simulink model "Vaja7b"  (R2013a)
settings: Solver=ode45  StartTime=0.0  StopTime=1  MaxStep=1e-4
undefined symbols (not defined in the file or in its folder): DiscIntNeverNeededParam
libraries: simulink x3
settings Model: Creator=Studenti  LastModifiedBy=Studenti
settings DataIOCC: SignalLoggingSaveFormat=ModelDataLogs
settings DebuggingCC: MaxConsecutiveZCsMsg=none  MultiTaskDSMMsg=warning  MultiTaskCondExecSysMsg=none  StrictBusMsg=None
settings RTWCC: IncludeERTFirstTime=on
settings GRTTargetCC: CodeReplacementLibrary=None  CPPClassGenCompliant=on

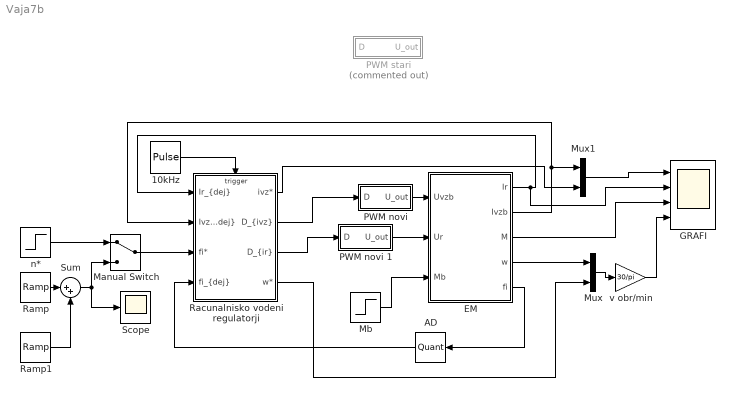
== system Vaja7b ==
  10kHz : DiscretePulseGenerator  PulseType=Time based  Period=1/10000  PulseWidth=5
  AD : Quantizer  QuantizationInterval=2*pi*2^-10
  EM : Subsystem  RequirementInfo="{}  %GIDa_e134c5b2_b96c_49ed_8b06_b6a8320c10d0"
  GRAFI : Scope  NumInputPorts=4
      settings: TimeRange=1  YMin=-4~0~-1~-100  YMax=4~0.5~1~300
  Manual Switch : ManualSwitch
  Mb : Step  Time=0.1  After=0.3  SampleTime=0
  Mux : Mux  Inputs=2
  Mux1 : Mux  Inputs=2
  "PWM novi " : Subsystem
  PWM novi 1 : Subsystem
  PWM stari : Subsystem  Commented=on
  Racunalnisko vodeni regulatorji : Subsystem
  Ramp : simulink/Sources/Ramp  slope=90*2*pi/60  start=0.1  X0=0
  Ramp1 : simulink/Sources/Ramp  slope=-90*2*pi/60  start=0.8  X0=0
  Scope : Scope
      settings: SaveName=ScopeData2
  Sum : Sum  Inputs=|++
  n* : Step  Time=0.2  After=pi*2  SampleTime=0
  v obr/min : Gain  Gain=30/pi
  wires:
  EM/3(M) -> GRAFI/3
  "PWM novi "/1(U_out) -> EM/1(Uvzb)
  PWM novi 1/1(U_out) -> EM/2(Ur)
  Mux/1 -> v obr/min/1
  Mb/1 -> EM/3(Mb)
  10kHz/1 -> Racunalnisko vodeni regulatorji/Trigger
  EM/2(Ivzb) -> Mux1/1, Racunalnisko vodeni regulatorji/2("Ivz_{dej}")
  Racunalnisko vodeni regulatorji/2("D_{ivz}") -> "PWM novi "/1(D)
  Racunalnisko vodeni regulatorji/1(ivz*) -> Mux1/2
  Racunalnisko vodeni regulatorji/3("D_{ir}") -> PWM novi 1/1(D)
  Racunalnisko vodeni regulatorji/4(w*) -> Mux/2
  EM/1(Ir) -> GRAFI/2, Racunalnisko vodeni regulatorji/1("Ir_{dej}")
  v obr/min/1 -> GRAFI/4
  EM/5(fi) -> AD/1
  AD/1 -> Racunalnisko vodeni regulatorji/4("fi_{dej}")
  EM/4(w) -> Mux/1
  Manual Switch/1 -> Racunalnisko vodeni regulatorji/3(fi*)
  n*/1 -> Manual Switch/1
  Ramp1/1 -> Sum/2
  Ramp/1 -> Sum/1
  Sum/1 -> Scope/1, Manual Switch/2
  Mux1/1 -> GRAFI/1

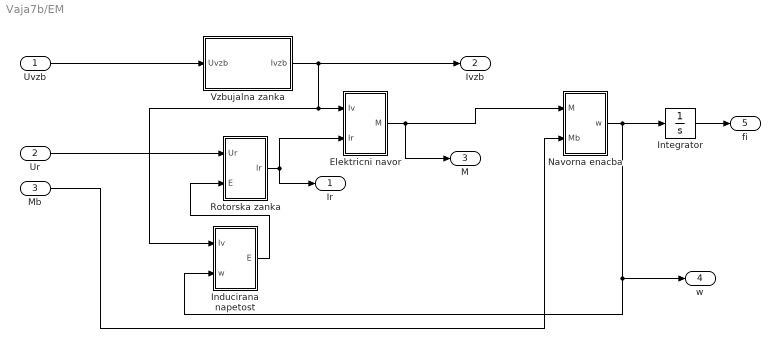
== system Vaja7b/EM ==
  Uvzb : Inport
  Ur : Inport  Port=2
  Mb : Inport  Port=3
  Elektricni navor : Subsystem
  Inducirana napetost : Subsystem
  Integrator : Integrator
  Navorna enacba : Subsystem
  Rotorska zanka : Subsystem
  Vzbujalna zanka : Subsystem
  Ir : Outport
  Ivzb : Outport  Port=2
  M : Outport  Port=3
  w : Outport  Port=4
  fi : Outport  Port=5
  wires:
  Uvzb/1 -> Vzbujalna zanka/1(Uvzb)
  Vzbujalna zanka/1(Ivzb) -> Ivzb/1, Inducirana napetost/1(Iv), Elektricni navor/1(Iv)
  Rotorska zanka/1(Ir) -> Elektricni navor/2(Ir), Ir/1
  Navorna enacba/1(w) -> w/1, Inducirana napetost/2(w), Integrator/1
  Elektricni navor/1(M) -> M/1, Navorna enacba/1(M)
  Inducirana napetost/1(E) -> Rotorska zanka/2(E)
  Ur/1 -> Rotorska zanka/1(Ur)
  Mb/1 -> Navorna enacba/2(Mb)
  Integrator/1 -> fi/1

== system Vaja7b/PWM novi  ==
  D : Inport
  Saturation : Saturate  UpperLimit=24  LowerLimit=-24
  Transfer Fcn : TransferFcn  Numerator=[24]  Denominator=[1/10000 1]
  U_out : Outport
  wires:
  Saturation/1 -> U_out/1
  Transfer Fcn/1 -> Saturation/1
  D/1 -> Transfer Fcn/1

== system Vaja7b/PWM novi 1 ==
  D : Inport
  Saturation : Saturate  UpperLimit=24  LowerLimit=-24
  Transfer Fcn : TransferFcn  Numerator=[24]  Denominator=[1/10000 1]
  U_out : Outport
  wires:
  Saturation/1 -> U_out/1
  Transfer Fcn/1 -> Saturation/1
  D/1 -> Transfer Fcn/1

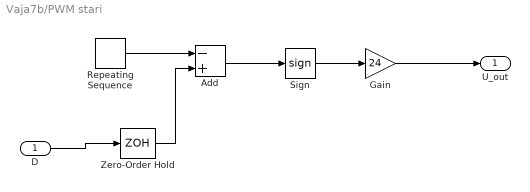
== system Vaja7b/PWM stari ==
  D : Inport
  Add : Sum  Inputs=-+
  Gain : Gain  Gain=24
  Repeating Sequence : simulink/Sources/Repeating Sequence  rep_seq_t=[0 0.0001]  rep_seq_y=[-1 1]
  Sign : Signum
  Zero-Order Hold : ZeroOrderHold  SampleTime=1/10000
  U_out : Outport
  wires:
  Gain/1 -> U_out/1
  Sign/1 -> Gain/1
  Repeating Sequence/1 -> Add/1
  Add/1 -> Sign/1
  Zero-Order Hold/1 -> Add/2
  D/1 -> Zero-Order Hold/1

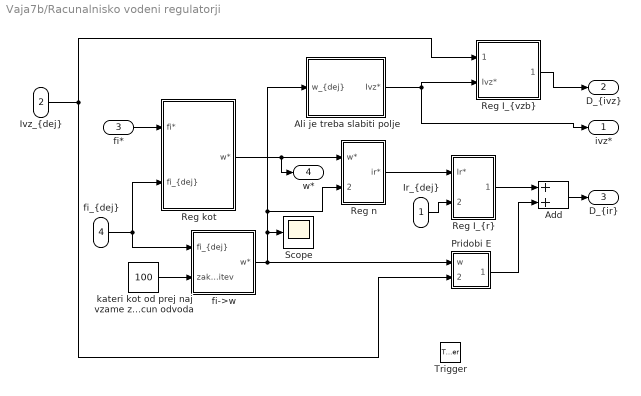
== system Vaja7b/Racunalnisko vodeni regulatorji ==
  "Ir_{dej}" : Inport
  "Ivz_{dej}" : Inport  Port=2
  fi* : Inport  Port=3
  "fi_{dej}" : Inport  Port=4
  Trigger : TriggerPort  PortDimensions=1
  Add : Sum
  Ali je treba slabiti polje : Subsystem
  Pridobi E : Subsystem
  "Reg I_{r}" : Subsystem
  "Reg I_{vzb}" : Subsystem
  Reg kot : Subsystem
  Reg n : Subsystem
  Scope : Scope
  fi->w : Subsystem
  kateri kot od prej naj vzame za izracun odvoda : Constant  Value=100
  ivz* : Outport
  "D_{ivz}" : Outport  Port=2
  "D_{ir}" : Outport  Port=3
  w* : Outport  Port=4
  wires:
  "Reg I_{r}"/1("D_{ir}") -> Add/1
  Reg n/1(ir*) -> "Reg I_{r}"/1(Ir*)
  "Reg I_{vzb}"/1("D_{ivz}") -> "D_{ivz}"/1
  Add/1 -> "D_{ir}"/1
  Ali je treba slabiti polje/1("Ivz* ") -> "Reg I_{vzb}"/2(Ivz*), ivz*/1
  Pridobi E/1(~E/24) -> Add/2
  Reg kot/1(w*) -> w*/1, Reg n/1(w*)
  "Ir_{dej}"/1 -> "Reg I_{r}"/2("Ir_{dej}")
  "Ivz_{dej}"/1 -> "Reg I_{vzb}"/1("Ivz_{dej}"), Pridobi E/2(Ivz)
  fi->w/1(w*) -> Scope/1, Ali je treba slabiti polje/1("w_{dej} "), Reg n/2("w_{dej}"), Pridobi E/1(w)
  "fi_{dej}"/1 -> fi->w/1("fi_{dej}"), Reg kot/2("fi_{dej}")
  kateri kot od prej naj vzame za izracun odvoda/1 -> fi->w/2(zakasnitev)
  fi*/1 -> Reg kot/1(fi*)

== system Vaja7b/EM/Elektricni navor ==
  Iv : Inport
  Ir : Inport  Port=2
  GQD : Gain  Gain=0.63
  Product : Product
  M : Outport
  wires:
  Ir/1 -> Product/2
  GQD/1 -> M/1
  Iv/1 -> Product/1
  Product/1 -> GQD/1

== system Vaja7b/EM/Inducirana napetost ==
  Iv : Inport
  w : Inport  Port=2
  GQD : Gain  Gain=0.63
  Product : Product
  E : Outport
  wires:
  Product/1 -> GQD/1
  Iv/1 -> Product/1
  w/1 -> Product/2
  GQD/1 -> E/1

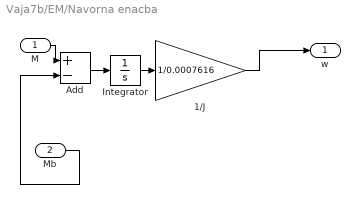
== system Vaja7b/EM/Navorna enacba ==
  M : Inport
  Mb : Inport  Port=2
  1/J : Gain  Gain=1/0.0007616
  Add : Sum  Inputs=+-
  Integrator : Integrator
  w : Outport
  wires:
  Integrator/1 -> 1/J/1
  1/J/1 -> w/1
  Add/1 -> Integrator/1
  M/1 -> Add/1
  Mb/1 -> Add/2

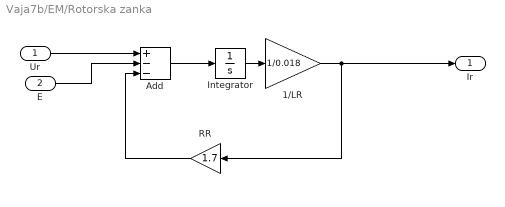
== system Vaja7b/EM/Rotorska zanka ==
  Ur : Inport
  E : Inport  Port=2
  1/LR : Gain  Gain=1/0.018
  Add : Sum  Inputs=+--
  Integrator : Integrator
  RR : Gain  Gain=1.7
  Ir : Outport
  wires:
  Add/1 -> Integrator/1
  Ur/1 -> Add/1
  RR/1 -> Add/3
  1/LR/1 -> RR/1, Ir/1
  Integrator/1 -> 1/LR/1
  E/1 -> Add/2

== system Vaja7b/EM/Vzbujalna zanka ==
  Uvzb : Inport
  1/Lv : Gain  Gain=1/4.01
  Integrator : Integrator
  Rv : Gain  Gain=25.8
  Sum : Sum  Inputs=|+-
  Ivzb : Outport
  wires:
  Rv/1 -> Sum/2
  Sum/1 -> Integrator/1
  Integrator/1 -> 1/Lv/1
  Uvzb/1 -> Sum/1
  1/Lv/1 -> Rv/1, Ivzb/1

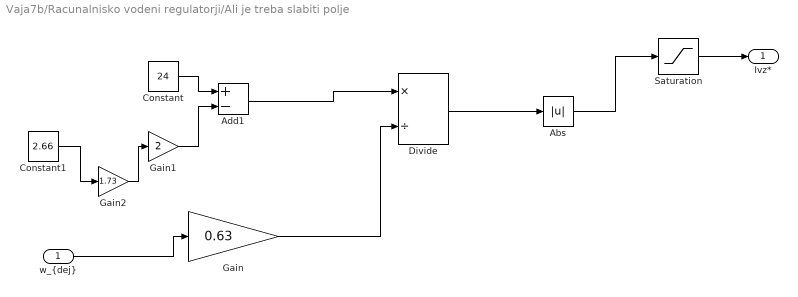
== system Vaja7b/Racunalnisko vodeni regulatorji/Ali je treba slabiti polje ==
  "w_{dej} " : Inport
  Abs : Abs
  Add1 : Sum  Inputs=+-
  Constant : Constant  Value=24
  Constant1 : Constant  Value=2.66
  Divide : Product  Inputs=*/
  Gain : Gain  Gain=0.63
  Gain1 : Gain  Gain=2
  Gain2 : Gain  Gain=1.73
  Saturation : Saturate  UpperLimit=0.48  LowerLimit=0
  "Ivz* " : Outport
  wires:
  Divide/1 -> Abs/1
  Saturation/1 -> "Ivz* "/1
  Gain1/1 -> Add1/2
  Abs/1 -> Saturation/1
  "w_{dej} "/1 -> Gain/1
  Gain/1 -> Divide/2
  Add1/1 -> Divide/1
  Constant/1 -> Add1/1
  Gain2/1 -> Gain1/1
  Constant1/1 -> Gain2/1

== system Vaja7b/Racunalnisko vodeni regulatorji/Pridobi E ==
  w : Inport
  Ivz : Inport  Port=2
  Divide : Product  Inputs=**
  Gain : Gain  Gain=0.63/24
  ~E/24 : Outport
  wires:
  Gain/1 -> ~E/24/1
  w/1 -> Divide/2
  Ivz/1 -> Divide/1
  Divide/1 -> Gain/1

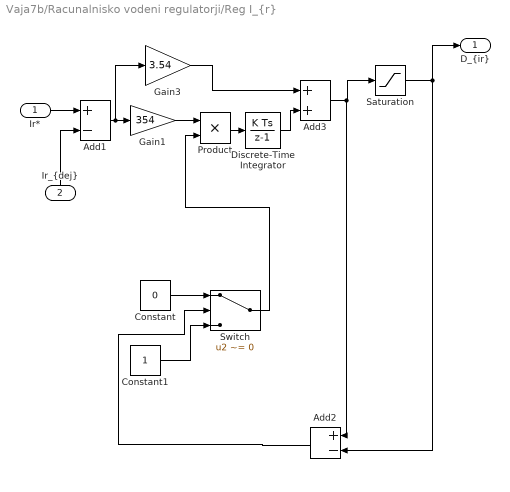
== system Vaja7b/Racunalnisko vodeni regulatorji/Reg I_{r} ==
  Ir* : Inport
  "Ir_{dej}" : Inport  Port=2
  Add1 : Sum  Inputs=+-
  Add2 : Sum  Inputs=+-
  Add3 : Sum
  Constant : Constant  Value=0
  Constant1 : Constant
  Discrete-Time Integrator : DiscreteIntegrator  SampleTime=-1  ICPrevOutput=DiscIntNeverNeededParam  ICPrevScaledInput=DiscIntNeverNeededParam
  Gain1 : Gain  Gain=354
  Gain3 : Gain  Gain=3.54
  Product : Product
  Saturation : Saturate  UpperLimit=1  LowerLimit=-1
  Switch : Switch  Criteria=u2 ~= 0  ZeroCross=off
  "D_{ir}" : Outport
  wires:
  Discrete-Time Integrator/1 -> Add3/2
  Gain3/1 -> Add3/1
  Add1/1 -> Gain1/1, Gain3/1
  "Ir_{dej}"/1 -> Add1/2
  Ir*/1 -> Add1/1
  Add3/1 -> Add2/1, Saturation/1
  Saturation/1 -> Add2/2, "D_{ir}"/1
  Switch/1 -> Product/2
  Constant/1 -> Switch/1
  Constant1/1 -> Switch/3
  Add2/1 -> Switch/2
  Gain1/1 -> Product/1
  Product/1 -> Discrete-Time Integrator/1

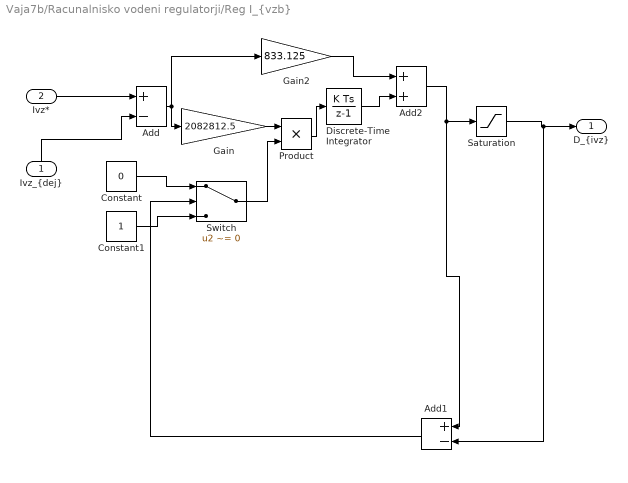
== system Vaja7b/Racunalnisko vodeni regulatorji/Reg I_{vzb} ==
  "Ivz_{dej}" : Inport
  Ivz* : Inport  Port=2
  Add : Sum  Inputs=+-
  Add1 : Sum  Inputs=+-
  Add2 : Sum
  Constant : Constant  Value=0
  Constant1 : Constant
  Discrete-Time Integrator : DiscreteIntegrator  SampleTime=-1  ICPrevOutput=DiscIntNeverNeededParam  ICPrevScaledInput=DiscIntNeverNeededParam
  Gain : Gain  Gain=2082812.5
  Gain2 : Gain  Gain=833.125
  Product : Product
  Saturation : Saturate  UpperLimit=1  LowerLimit=-1
  Switch : Switch  Criteria=u2 ~= 0  ZeroCross=off
  "D_{ivz}" : Outport
  wires:
  Discrete-Time Integrator/1 -> Add2/2
  Gain2/1 -> Add2/1
  Ivz*/1 -> Add/1
  Add/1 -> Gain/1, Gain2/1
  "Ivz_{dej}"/1 -> Add/2
  Add2/1 -> Saturation/1, Add1/1
  Switch/1 -> Product/2
  Constant/1 -> Switch/1
  Constant1/1 -> Switch/3
  Add1/1 -> Switch/2
  Saturation/1 -> Add1/2, "D_{ivz}"/1
  Gain/1 -> Product/1
  Product/1 -> Discrete-Time Integrator/1

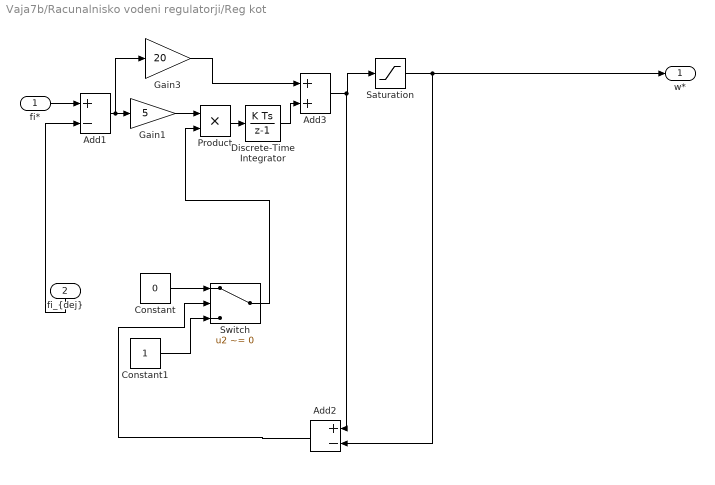
== system Vaja7b/Racunalnisko vodeni regulatorji/Reg kot ==
  fi* : Inport
  "fi_{dej}" : Inport  Port=2
  Add1 : Sum  Inputs=+-
  Add2 : Sum  Inputs=+-
  Add3 : Sum
  Constant : Constant  Value=0
  Constant1 : Constant
  Discrete-Time Integrator : DiscreteIntegrator  SampleTime=-1  ICPrevOutput=DiscIntNeverNeededParam  ICPrevScaledInput=DiscIntNeverNeededParam
  Gain1 : Gain  Gain=5
  Gain3 : Gain  Gain=20
  Product : Product
  Saturation : Saturate  UpperLimit=1000*2*pi/60  LowerLimit=-1000*2*pi/60
  Switch : Switch  Criteria=u2 ~= 0  ZeroCross=off
  w* : Outport
  wires:
  Discrete-Time Integrator/1 -> Add3/2
  Gain3/1 -> Add3/1
  Add1/1 -> Gain1/1, Gain3/1
  "fi_{dej}"/1 -> Add1/2
  fi*/1 -> Add1/1
  Add3/1 -> Add2/1, Saturation/1
  Switch/1 -> Product/2
  Constant/1 -> Switch/1
  Constant1/1 -> Switch/3
  Add2/1 -> Switch/2
  Gain1/1 -> Product/1
  Product/1 -> Discrete-Time Integrator/1
  Saturation/1 -> Add2/2, w*/1

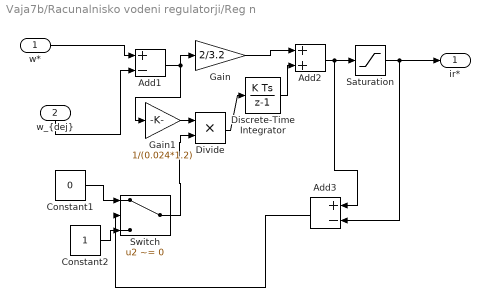
== system Vaja7b/Racunalnisko vodeni regulatorji/Reg n ==
  w* : Inport
  "w_{dej}" : Inport  Port=2
  Add1 : Sum  Inputs=+-
  Add2 : Sum
  Add3 : Sum  Inputs=+-
  Constant1 : Constant  Value=0
  Constant2 : Constant
  Discrete-Time Integrator : DiscreteIntegrator  SampleTime=-1  ICPrevOutput=DiscIntNeverNeededParam  ICPrevScaledInput=DiscIntNeverNeededParam
  Divide : Product  Inputs=**
  Gain : Gain  Gain=2/3.2
  Gain1 : Gain  Gain=1/(0.024*1.2)
  Saturation : Saturate  UpperLimit=2.66  LowerLimit=-2.66
  Switch : Switch  Criteria=u2 ~= 0  ZeroCross=off
  ir* : Outport
  wires:
  "w_{dej}"/1 -> Add1/2
  Gain/1 -> Add2/1
  Add1/1 -> Gain1/1, Gain/1
  Discrete-Time Integrator/1 -> Add2/2
  w*/1 -> Add1/1
  Divide/1 -> Discrete-Time Integrator/1
  Gain1/1 -> Divide/1
  Saturation/1 -> Add3/2, ir*/1
  Add2/1 -> Add3/1, Saturation/1
  Switch/1 -> Divide/2
  Constant1/1 -> Switch/1
  Constant2/1 -> Switch/3
  Add3/1 -> Switch/2

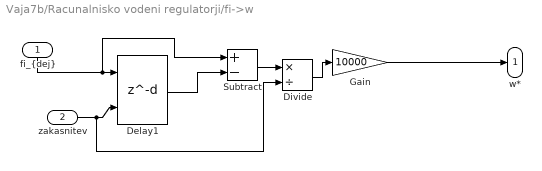
== system Vaja7b/Racunalnisko vodeni regulatorji/fi->w ==
  "fi_{dej}" : Inport
  zakasnitev : Inport  Port=2
  Delay1 : Delay  DelayLengthSource=Input port  DelayLength=10
      settings: InputPortMap=u0,p1
  Divide : Product  Inputs=*/
  Gain : Gain  Gain=10000
  Subtract : Sum  Inputs=+-
  w* : Outport
  wires:
  "fi_{dej}"/1 -> Subtract/1, Delay1/1
  Subtract/1 -> Divide/1
  Delay1/1 -> Subtract/2
  Gain/1 -> w*/1
  Divide/1 -> Gain/1
  zakasnitev/1 -> Divide/2, Delay1/2
